simulink model "ES200A_CurrMeas"  (R2013b)
settings: Solver=FixedStepDiscrete  SolverMode=SingleTasking  StartTime=0.0  StopTime=1  FixedStep=0.000125  RelTol=1e-3
undefined symbols (not defined in the file): ARCHGLBPRM_2PI_ULS_F32, CurrMeasEolGainMax, CurrMeasEolGainMin, CurrMeasEolGainNrOfSample, CurrMeasEolGainNumer, CurrMeasEolMaxMotVel, CurrMeasEolOffsHiBrdgVltgMin, CurrMeasEolOffsHiCmuOffs, CurrMeasEolOffsLoCmuOffs, CurrMeasEolOffsMax, CurrMeasEolOffsMin, CurrMeasEolOffsNrOfSample, CurrMeasEolTranCntrThd, CurrMeasMinRqrdPhaOnTi, CurrMeasMotAgCompuDly, CurrMeasMotCurrAdcVlyWrmIninMax, CurrMeasMotCurrAdcVlyWrmIninMin, CurrMeasNtc0x05DFailStep, CurrMeasNtc0x05DPassStep, CurrMeasNtc0x06DFailStep, CurrMeasNtc0x06DPassStep, DEGREES30_MOTRAD_F32, DIFOFFSRNGCHKMAX_VOLT_F32, ELECGLBPRM_IVTRCNT_CNT_U08, ELECGLBPRM_STRTUPSTCURRMEASWRMININTESTSTRT_CNT_U08, FLTINJ_CURRMEAS_MOTCURRCORRDA, FLTINJ_CURRMEAS_MOTCURRCORRDD, FLTINJ_CURRMEAS_TESTOK, MAXCURRCORRD_AMPR_F32, PhaABCMeasdOutOfRng, PhaDEFMeasOutOfRng, SysGlbPrmMotPoleCnt
libraries: simulink x10, FixdToFloat x1
(part 1 of 7)
settings Model: NumberOfSteps=100  Creator=hzy4g9  LastModifiedBy=wzvp6q
settings SolverCC: AutoInsertRateTranBlk=on  InsertRTBMode=Always
settings DataIOCC: LimitDataPoints=off  SaveFormat=Structure  ReturnWorkspaceOutputs=on
settings OptimizationCC: BlockReduction=off  InlineParams=on  ZeroExternalMemoryAtStartup=off  ZeroInternalMemoryAtStartup=off  OptimizeModelRefInitCode=on  LifeSpan=1
settings DebuggingCC: SignalInfNanChecking=error  SignalRangeChecking=warning  UnderspecifiedInitializationDetection=Simplified  SolverPrmCheckMsg=error  InheritedTsInSrcMsg=error  DiscreteInheritContinuousMsg=error  SingleTaskRateTransMsg=error  TasksWithSamePriorityMsg=error  SigSpecEnsureSampleTimeMsg=error  CheckMatrixSingularityMsg=error  ParameterUnderflowMsg=error  ParameterPrecisionLossMsg=error  ParameterTunabilityLossMsg=error  FixptConstUnderflowMsg=warning  FixptConstOverflowMsg=warning  VectorMatrixConversionMsg=error  SignalLabelMismatchMsg=error  UnconnectedInputMsg=error  UnconnectedOutputMsg=error  UnconnectedLineMsg=error  SFcnCompatibilityMsg=error  UniqueDataStoreMsg=warning  BusObjectLabelMismatch=error  RootOutportRequireBusObject=error  AssertControl=DisableAll  ModelReferenceIOMsg=error  ModelReferenceVersionMismatchMessage=warning  ModelReferenceIOMismatchMessage=error  ModelReferenceCSMismatchMessage=warning  ModelReferenceDataLoggingMessage=error  StateNameClashWarn=warning  StrictBusMsg=ErrorOnBusTreatedAsVector  NonBusSignalsTreatedAsBus=error  SFUnusedDataAndEventsDiag=none  SFUnexpectedBacktrackingDiag=error  SFInvalidInputDataAccessInChartInitDiag=error  SFNoUnconditionalDefaultTransitionDiag=error  SFTransitionOutsideNaturalParentDiag=error  SFUnconditionalTransitionShadowingDiag=error  SFUndirectedBroadcastEventsDiag=error
settings ModelReferenceCC: ModelReferenceNumInstancesAllowed=Single
settings RTWCC: SystemTargetFile=autosar.tlc  GenCodeOnly=on  TemplateMakefile=ert_default_tmf  Description=AUTOSAR  GenerateReport=on  ProcessScript=autosar_make_rtw_hook  LaunchReport=on
settings CodeAppCC: GenerateComments=off  IgnoreCustomStorageClasses=off  CustomSymbolStrType=$N$R$M  CustomSymbolStrBlkIO=$N$M  SimulinkBlockComments=off
settings STFCustomTargetCC: ParMdlRefBuildCompliant=on  CompOptLevelCompliant=on  IncludeMdlTerminateFcn=off  CombineOutputUpdateFcns=on  SuppressErrorStatus=on  ERTFirstTimeCompliant=on  ERTCustomFileBanners=on  SupportNonFinite=off  SupportComplex=off  SupportContinuousTime=off  SupportNonInlinedSFcns=off  MATLABClassNameForMDSCustomization=Simulink.SoftwareTarget.ERTCustomization  AutosarCompliant=on  GRTInterface=off  SystemTargetFile=autosar.tlc
settings ERTTargetCC: CodeReplacementLibrary=ANSI_C  ConcurrentExecutionCompliant=off  IncludeMdlTerminateFcn=off  SuppressErrorStatus=on  SupportNonFinite=off  SupportComplex=off  ModelStepFunctionPrototypeControlCompliant=off  CPPClassGenCompliant=off  AutosarCompliant=on  InlinedParameterPlacement=NonHierarchical  ERTCustomFileTemplate=example_file_process.tlc  EnableUserReplacementTypes=on

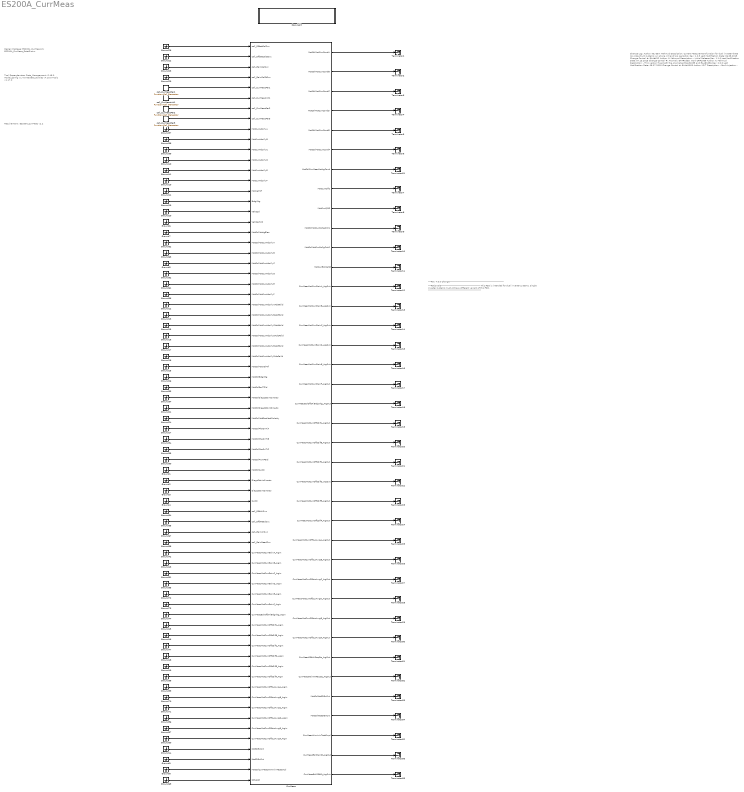
== system ES200A_CurrMeas ==
  note: ***Rev 4.6.0 Change******************************************************
  note: ***Rationale***************************************
      | This FDD is intended for dual inverter systems.
      | Single inverter systems must utilize a different
      | variant of this FDD.
      | *****************************************************
  note: Change Log:
      |
      | Author: Nayeem Mahmud
      | Description:
      | Current Measurement function for dual inverter three low side shunt systems run at one init and two periodics.
      |
      | Rev: 1.0.3
      | Last Modification Date: 06.08.2015
      | Change Control #: EA4#612
      | Author: N. Mahmud
      | Description:
      | - Initial Release
      |
      |
      | Rev: 1.1.0
      | Last Modification Date: 07.13.2015
      | Change Control #: Anomaly EA4#1035, Work CR#1068
      | Author: N. Mahmud
      | Description:
      | - This version fixes both the Anomalies EA4#1035 and EA4#1036
      |
      | Rev: 2.0.0
      | Last Modification Date: 08.07.2015
      | Change Control #: EA4#1003
      | Author: KPIT
      | Description:
      | - Fault Injection blocks added for output MotCtrlMotCurrCorrdA, MotCtrlMotCurrCorrdD and RangeCheckENABC
      |
      | Rev: 2.0.1
      | Last Modification Date: 08.12.2015
      | Change Control #: EA4#1268
      | Author: KPIT
      | Description:
      | - Renamed Fault Injection blocks for output MotCtrlMotCurrCorrdA, MotCtrlMotCurrCorrdD and RangeCheckENABC
      |
      |
      | Rev: 3.0.0
      | Last Modification Date: 09.25.2015
      | Change Control #: Anomaly # 1662, Work CR#1666
      | Author: N. Mahmud
      | Description:
      | - Added a new 2ms periodic - SetNtcSt and GetQlfrSt functions and Warm Init Test are moved into the new 2ms periodic.
      | - Multiple variable names (PIMs, NVMs, etc) have been updated according to the naming convention.
      | - NVM structure with 19 elements has been divided into two structures for Offset (13 elements) and Gain (6 elements).
      | - CurrMeasGainReadReq, CurrMeasGainWrReq, CurrMeasOffsReadReq, CurrMeasOffsWrReq Server functions have been added.
      |
      | Rev: 3.1.0
      | Last Modification Date: 10.01.2015
      | Change Control #: Anomaly # 1662, Work CR#1786
      | DRW: N. Mahmud
      | Description:
      | - Fixed the m file naming mismatch
      | - Changed some logic in the EOL gain and Offset Service
      |
      |
      | Rev: 3.2.0
      | Last Modification Date: 10.20.2015
      | Change Control #: Anomaly # 1784, Component CR # 2048, Work CR#2052
      | DRW: N. Mahmud
      | Description:
      | - Added the parameter bytes for warm Init, Enable - protocol check
      | - Corrected some input/oputput issues in the m file
      | - Corrected some requirement linkage issues
      |
      |
      | Rev: 4.0.0
      | Last Modification Date: 11.06.2015
      | Change Control #: Anomaly # 2171 + ICR 2398, Component CR # 2297, Work CR#2317
      | Author: N. Mahmud
      | Description:
      | - Fixed Anomaly # 2171: Two response returns were added - one is "Offset Write Request Status" and another one is "Gain Write Request Status". They will be function output arguments.
      | - ICR 2398: EolOffsSts and EolGainSts values were added to cover the full range of faults that will be translated into "Negative Response Codes"
      | - CurrMeasEolOffsStReq and CurrMeasEolGainStReq has been change to CurrMeasEolOffsStsReq and CurrMeasEolGainStsReq
      |
      |
      | Rev: 4.1.0
      | Last Modified Date: 24-12-2015
      | Change Control #:  EA4#3977
      | Author: Hari Prasad(KPIT)
      | Description:
      | - Resolved simulation issues
      | - Adc Failed inputs and logic related to it has been added
      | - Following calibrations have been deleted
      | CurrMeasMotCurrAdcVlyEnadMin, CurrMeasMotCurrAdcVlyEnadMax
      | - Callibration 'CurrMeasMinRqrdPhaOnTi' has been updated
      |
      | Rev: 4.2.0
      | Last Modified Date: 03.29.2016
      | Change Control #:  Component EA4#3881, Work CR#4988
      | Author: Nayeem Mahmud
      | Description:
      | - Model update to match with the code/optomization:
      | 	- Per_2: Function:	1. "CalcMotCurrMotAgCorrd()" should not be called when the first condition check is failed.
      | 			2. Remove the MotCtrlDiagcStsIvtr(1/2)Inactv check everytime when calculating the correct currents
      | 			3. Move the Offset Calc ABC/DEF just after when the ProtocolChkEn passes
      | 	- Per_1: Offset: 	1. In case 0/1 "CurrMeasEolAvrgCntr" should be implemented properly.
      | 			2. Remove the extra 6 condition check.
      | 			3. Two pass_step/fail_step cal can be removed.
      | 	- Per_1: Gain:	1. Update the very first condition check.
      | 			2. Two pass_step/fail_step cal can be removed.
      |
      |
      | Rev: 4.3.0
      | Last Modified Date: 07.18.2016
      | Change Control #:  Work CR#6615
      | Author: Gerald McCann
      | Description:
      | - Model update for Unit Test:
      | 	1) Update ranges on PIM (See Anomaly EA4#5895)
      | 	2) Various updates for MIL (See Anomaly EA4#6428)
      | - Add rollover compensation to MotCtrlCurrMeasMotAgCorrd for values outside its current range of +/-2pi
      | - Removed 8 physical inputs MotCurrInpPhyA, MotCurrInpPhyB, MotCurrInpPhyC, MotCurrInpPhyD, MotCurrInpPhyE, MotCurrInpPhyF, MotCurrSnsrOffs1, MotCurrSnsrOffs2
      | - Remove DataStoreMemory blocks for MotCurrEolOffsDifA, MotCurrEolOffsDifB, MotCurrEolOffsDifC, MotCurrEolOffsDifD, MotCurrEolOffsDifE, MotCurrEolOffsDifF
      | - Add NVM CurrMeasEolOffsCalSet DataStoreRead in CurrMeasInit1
      | - Changed name of CurrMeasEolOffsSts to CurrMeasEolOffsSt to match .m file
      |
      |
      | Rev: 4.4.0
      | Last Modified Date: 08.02.2016
      | Change Control #:  Work CR#6727
      | Author: Gerald McCann
      | Description:
      | - Replace use of 2*pi with ARCHGLBPRM_2PI_ULS_F32
      |
      |
      | Rev: 4.5.0
      | Last Modified Date: 09.30.2016
      | Change Control #:  Work CR#7759
      | Author: Gerald McCann
      | Description:
      | - Add design rationale to Chart 1 in CurrMeasPer2
      | - Replace divisor CurrMeasEolGainNrOfSample with CurrMeasEolAvrgCntr in CurrMeasPer1 GainStateMachine. No functional impact.
      |
      |
      | Rev: 4.6.0
      | Last Modified Date: 11.07.2016
      | Change Control #:  Work CR#8298
      | Author: Gerald McCann
      | Description:
      | - In CurrMeasPer1, change both the offset and gain calibration functions to set OffsRngChkABC and GainRngChkABC to 0 if DiagcStsIvtr1Inactv is TRUE
      | - In CurrMeasPer1, change both the offset and gain calibration functions to set OffsRngChkDEF and GainRngChkDEF to 0 if DiagcStsIvtr2Inactv is TRUE
      | - In CurrMeasPer2, replace 'greater than' with 'greater than or equal to' in MotCtrlPhaOnTi checks
      | - Add rationale explaining this FDD is intended for dual inverter systems.  Single inverter systems must utilize a different variant of this FDD.
  note: Design Package:
      |
      | ES200A_CurrMeas.slx
      | ES200A_CurrMeas_DataDict.m
  note: Tool Dependancies:
      |
      | Data_Management v2.48.0
      | Model_Config v1.4.0
      | Nexteer_Utilities v4.10.0
      | Tools v1.17.0
  note: Requirement :
      |
      | ES200A_CurrMeas v2.2
  Copyright : Subsystem  Description=|  mask(Copyright Information){none=on}
      | Copyright info block.                                               
      |                                                                     
      | Place copyright information at the top of every subsystem in design.
      mask prompts: none "No parameters"
      mask help: Place copyright information at the top of every subsystem in design.
      mask Display:
      | NxtrConf = 'Nexteer Confidential';
      | 
      | sys = bdroot; %handle for the current model ("system")
      | first = get_param(sys,'Created');
      | if(isempty(first))
      |     first = datestr(now,'yyyy');
      | else
      |     first = first(end-3:end);  %year is last four digits
      | end
      | 
      | last = get_param(sys,'LastModifiedDate');
      | if isempty(last)
      |     last = datestr(now,'yyyy');
      | else
      |     last = last(end-3:end);
      | end
      | 
      | if strcmp(first,last)
      |     fprintf('%s\nCopyright  %s Nexteer',NxtrConf,first);
      | else
      |     fprintf('%s\n%s%s-%s Nexteer',NxtrConf,char(169),first,last);
      | end
  CurrMeas : Subsystem  RequirementInfo={'linktype_rmi_doors' '000089bc (/ESG Group/FDD Module Requirements/EA4 Specific/ES200A_CurrMeas)' '#ES200A_15' 'true' 'REQ: ES200A_15' '' } %GIDa_3da50868_19fe_4888_8a05_c6ca52f8a06e
  Ground{1..29,34..35,37..73} (68 alike) : Ground
  Terminator{1..36,51..52} (38 alike) : Terminator
  call_CurrMeasInit1 : simulink/Ports & Subsystems/Function-Call Generator  sample_time=0  numberOfIterations=1
  call_CurrMeasPer1 : simulink/Ports & Subsystems/Function-Call Generator  sample_time=.002  numberOfIterations=1
  call_CurrMeasPer2 : simulink/Ports & Subsystems/Function-Call Generator  sample_time=.000125  numberOfIterations=1
  call_CurrMeasPer3 : simulink/Ports & Subsystems/Function-Call Generator  sample_time=.002  numberOfIterations=1
  wires:
  CurrMeas/13(CurrMeasMotCurrGainA_ArgOut) -> Terminator12/1
  CurrMeas/14(CurrMeasMotCurrGainB_ArgOut) -> Terminator13/1
  CurrMeas/15(CurrMeasMotCurrGainC_ArgOut) -> Terminator14/1
  CurrMeas/16(CurrMeasMotCurrGainD_ArgOut) -> Terminator15/1
  CurrMeas/17(CurrMeasMotCurrGainE_ArgOut) -> Terminator16/1
  CurrMeas/18(CurrMeasMotCurrGainF_ArgOut) -> Terminator17/1
  CurrMeas/19(CurrMeasEolOffsHiBrdgVltg_ArgOut) -> Terminator18/1
  CurrMeas/20(CurrMeasMotCurrOffsDifA_ArgOut) -> Terminator19/1
  CurrMeas/21(CurrMeasMotCurrOffsDifB_ArgOut) -> Terminator20/1
  CurrMeas/22(CurrMeasMotCurrOffsDifC_ArgOut) -> Terminator21/1
  CurrMeas/23(CurrMeasMotCurrOffsDifD_ArgOut) -> Terminator22/1
  CurrMeas/24(CurrMeasMotCurrOffsDifE_ArgOut) -> Terminator23/1
  CurrMeas/25(CurrMeasMotCurrOffsDifF_ArgOut) -> Terminator24/1
  CurrMeas/26(CurrMeasMotCurrOffsLoAvrgA_ArgOut) -> Terminator25/1
  CurrMeas/27(CurrMeasMotCurrOffsLoAvrgB_ArgOut) -> Terminator26/1
  CurrMeas/28(CurrMeasMotCurrOffsLoAvrgC_ArgOut) -> Terminator27/1
  CurrMeas/29(CurrMeasMotCurrOffsLoAvrgD_ArgOut) -> Terminator28/1
  CurrMeas/30(CurrMeasMotCurrOffsLoAvrgE_ArgOut) -> Terminator29/1
  CurrMeas/31(CurrMeasMotCurrOffsLoAvrgF_ArgOut) -> Terminator30/1
  CurrMeas/32(CurrMeasOffsWrReqSts_ArgOut) -> Terminator51/1
  CurrMeas/33(CurrMeasGainWrReqSts_ArgOut) -> Terminator52/1
  Ground29/1 -> CurrMeas/4(call_GainCalStSvc)
  Ground23/1 -> CurrMeas/3(call_GainCalSvc)
  Ground22/1 -> CurrMeas/2(call_OffsetCalStSvc)
  Ground28/1 -> CurrMeas/1(call_OffsetCalSvc)
  call_CurrMeasPer1/1 -> CurrMeas/5(call_CurrMeasPer1)
  call_CurrMeasInit1/1 -> CurrMeas/6(call_CurrMeasInit1)
  call_CurrMeasPer2/1 -> CurrMeas/7(call_CurrMeasPer2)
  call_CurrMeasPer3/1 -> CurrMeas/8(call_CurrMeasPer3)
  Ground37/1 -> CurrMeas/9(MotCurrAdcVlyA)
  Ground38/1 -> CurrMeas/10(MotCurrAdcVlyB)
  Ground39/1 -> CurrMeas/11(MotCurrAdcVlyC)
  Ground40/1 -> CurrMeas/12(MotCurrAdcVlyD)
  Ground41/1 -> CurrMeas/13(MotCurrAdcVlyE)
  Ground10/1 -> CurrMeas/14(MotCurrAdcVlyF)
  Ground53/1 -> CurrMeas/34(MotCtrlEcuTFild)
  Ground54/1 -> CurrMeas/35(MotCtrlDiagcStsIvtr1Inactv)
  Ground6/1 -> CurrMeas/18(VehSpdVld)
  Ground7/1 -> CurrMeas/19(MotCtrlMotAgElec)
  Ground19/1 -> CurrMeas/16(BrdgVltg)
  Ground25/1 -> CurrMeas/32(MotCtrlMotVelMrf)
  Ground17/1 -> CurrMeas/30(MotCtrlMotCurrAdcVlyEAdcFaild)
  Ground12/1 -> CurrMeas/26(MotCtrlMotCurrAdcVlyAAdcFaild)
  Ground21/1 -> CurrMeas/36(MotCtrlDiagcStsIvtr2Inactv)
  Ground18/1 -> CurrMeas/31(MotCtrlMotCurrAdcVlyFAdcFaild)
  Ground15/1 -> CurrMeas/28(MotCtrlMotCurrAdcVlyCAdcFaild)
  Ground20/1 -> CurrMeas/17(VehSpd)
  Ground26/1 -> CurrMeas/33(MotCtrlBrdgVltg)
  Ground27/1 -> CurrMeas/38(MotCtrlPhaOnTiA)
  Ground11/1 -> CurrMeas/15(MotVelMrf)
  Ground24/1 -> CurrMeas/37(MotCtrlMotElecMeclPolarity)
  Ground13/1 -> CurrMeas/27(MotCtrlMotCurrAdcVlyBAdcFaild)
  Ground16/1 -> CurrMeas/29(MotCtrlMotCurrAdcVlyDAdcFaild)
  Ground34/1 -> CurrMeas/39(MotCtrlPhaOnTiB)
  Ground35/1 -> CurrMeas/40(MotCtrlPhaOnTiC)
  Ground4/1 -> CurrMeas/45(SysSt)
  Ground42/1 -> CurrMeas/50(CurrMeasMotCurrGainA_ArgIn)
  Ground43/1 -> CurrMeas/51(CurrMeasMotCurrGainB_ArgIn)
  Ground44/1 -> CurrMeas/56(CurrMeasEolOffsHiBrdgVltg_ArgIn)
  Ground45/1 -> CurrMeas/57(CurrMeasMotCurrOffsDifA_ArgIn)
  Ground46/1 -> CurrMeas/58(CurrMeasMotCurrOffsDifB_ArgIn)
  Ground47/1 -> CurrMeas/59(CurrMeasMotCurrOffsDifC_ArgIn)
  Ground48/1 -> CurrMeas/60(CurrMeasMotCurrOffsDifD_ArgIn)
  Ground49/1 -> CurrMeas/61(CurrMeasMotCurrOffsDifE_ArgIn)
  Ground50/1 -> CurrMeas/41(MotCtrlPwmPerd)
  Ground51/1 -> CurrMeas/52(CurrMeasMotCurrGainC_ArgIn)
  Ground55/1 -> CurrMeas/53(CurrMeasMotCurrGainD_ArgIn)
  Ground58/1 -> CurrMeas/62(CurrMeasMotCurrOffsDifF_ArgIn)
  Ground59/1 -> CurrMeas/63(CurrMeasMotCurrOffsLoAvrgA_ArgIn)
  Ground64/1 -> CurrMeas/46(call_OffsWrSvc)
  Ground65/1 -> CurrMeas/47(call_OffsReadSvc)
  Ground67/1 -> CurrMeas/48(call_GainWrSvc)
  Ground68/1 -> CurrMeas/49(call_GainReadSvc)
  Ground72/1 -> CurrMeas/54(CurrMeasMotCurrGainE_ArgIn)
  Ground73/1 -> CurrMeas/55(CurrMeasMotCurrGainF_ArgIn)
  Ground2/1 -> CurrMeas/43(DiagcStsIvtr1Inactv)
  Ground3/1 -> CurrMeas/44(DiagcStsIvtr2Inactv)
  Ground1/1 -> CurrMeas/42(MotCtrlSysSt)
  CurrMeas/2(MotCtrlMotCurrCorrdB) -> Terminator2/1
  CurrMeas/1(MotCtrlMotCurrCorrdA) -> Terminator1/1
  CurrMeas/3(MotCtrlMotCurrCorrdC) -> Terminator3/1
  CurrMeas/4(MotCtrlMotCurrCorrdD) -> Terminator4/1
  CurrMeas/5(MotCtrlMotCurrCorrdE) -> Terminator5/1
  CurrMeas/6(MotCtrlMotCurrCorrdF) -> Terminator6/1
  CurrMeas/8(MotCurrQlfr1) -> Terminator7/1
  CurrMeas/9(MotCurrQlfr2) -> Terminator8/1
  CurrMeas/10(MotCtrlMotCurrRollgCntr1) -> Terminator9/1
  CurrMeas/11(MotCtrlMotCurrRollgCntr2) -> Terminator10/1
  CurrMeas/12(MotCurrEolCalSt) -> Terminator11/1
  CurrMeas/7(MotCtrlCurrMeasMotAgCorrd) -> Terminator31/1
  Ground62/1 -> CurrMeas/20(MotCtrlMotCurrAdcVlyA)
  Ground63/1 -> CurrMeas/21(MotCtrlMotCurrAdcVlyB)
  Ground61/1 -> CurrMeas/24(MotCtrlMotCurrAdcVlyE)
  Ground5/1 -> CurrMeas/22(MotCtrlMotCurrAdcVlyC)
  Ground66/1 -> CurrMeas/25(MotCtrlMotCurrAdcVlyF)
  Ground52/1 -> CurrMeas/23(MotCtrlMotCurrAdcVlyD)
  Ground60/1 -> CurrMeas/68(CurrMeasMotCurrOffsLoAvrgF_ArgIn)
  Ground70/1 -> CurrMeas/64(CurrMeasMotCurrOffsLoAvrgB_ArgIn)
  Ground57/1 -> CurrMeas/67(CurrMeasMotCurrOffsLoAvrgE_ArgIn)
  Ground71/1 -> CurrMeas/65(CurrMeasMotCurrOffsLoAvrgC_ArgIn)
  Ground56/1 -> CurrMeas/66(CurrMeasMotCurrOffsLoAvrgD_ArgIn)
  Ground69/1 -> CurrMeas/72(StrtUpSt)
  Ground8/1 -> CurrMeas/71(MotCtrlCurrMeasWrmIninTestCmpl)
  CurrMeas/36(CurrMeasWrmIninTestCmpl) -> Terminator32/1
  Ground14/1 -> CurrMeas/69(Ntc5DErrCnt)
  Ground9/1 -> CurrMeas/70(Ntc6DErrCnt)
  CurrMeas/34(MotCtrlNtc5DErrCnt) -> Terminator33/1
  CurrMeas/35(MotCtrlNtc6DErrCnt) -> Terminator34/1
  CurrMeas/37(CurrMeasEolGainSt_ArgOut) -> Terminator36/1
  CurrMeas/38(CurrMeasEolOffsSt_ArgOut) -> Terminator35/1

== system ES200A_CurrMeas/Copyright ==
